simulink model "lf"  (Simulink 8.1)
settings: Solver=ode45  StartTime=0.0  StopTime=10.0  RelTol=1e-3
values from neighbouring files (symbols this model uses):
  A2 = 1.82742    [lf_param.m]
  A3 = 0.827764    [lf_param.m]
  B1 = 2.74759    [lf_param.m]
  B2 = 2.70322    [lf_param.m]
  fs = sq_wave_freq*osr    (= 10000)    [param2.m]
settings Model: Creator=amr  LastModifiedBy=amr
settings DataIOCC: SignalLoggingSaveFormat=Dataset
settings OptimizationCC: ExpressionDepthLimit=128
settings DebuggingCC: FcnCallInpInsideContextMsg=EnableAllAsError
settings GRTTargetCC: CombineOutputUpdateFcns=on  GRTInterface=off

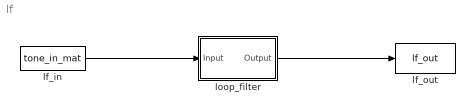
== system lf ==
  lf_in : FromWorkspace  VariableName=tone_in_mat  OutDataTypeStr=fixdt(1,16,15)  SampleTime=1/fs  Interpolate=off  OutputAfterFinalValue=Holding final value
  lf_out : ToWorkspace  VariableName=lf_out  SampleTime=-1
  loop_filter : Subsystem  Tag=FilterWizardSubSystem
      settings: ErrorFcn=dspFilterRealizedInBasicElemsAlgLoopErrFcnCallback
  wires:
  lf_in/1 -> loop_filter/1(Input)
  loop_filter/1(Output) -> lf_out/1

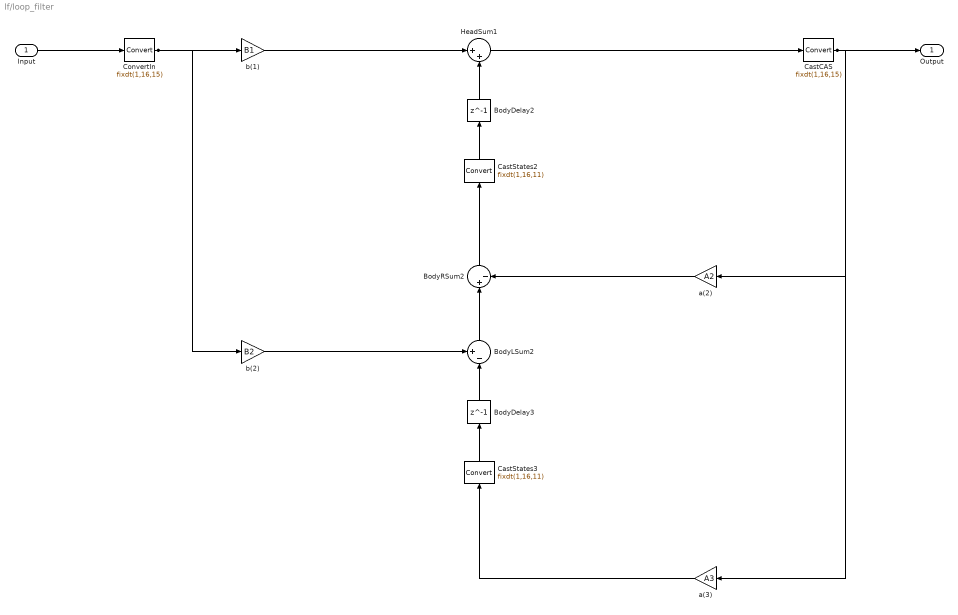
== system lf/loop_filter ==
  Input : Inport
  BodyDelay2 : Delay  DelayLength=1  InitialCondition=0
  BodyDelay3 : Delay  DelayLength=1  InitialCondition=0
  BodyLSum2 : Sum  Inputs=+-|  AccumDataTypeStr=fixdt(1,35,30)  OutDataTypeStr=fixdt(1,25,20)  SaturateOnIntegerOverflow=on
  BodyRSum2 : Sum  Inputs=|+-  AccumDataTypeStr=fixdt(1,35,30)  OutDataTypeStr=fixdt(1,25,20)  SaturateOnIntegerOverflow=on
  CastCAS : DataTypeConversion  OutDataTypeStr=fixdt(1,16,15)  SaturateOnIntegerOverflow=on
  CastStates2 : DataTypeConversion  OutDataTypeStr=fixdt(1,16,11)  SaturateOnIntegerOverflow=on
  CastStates3 : DataTypeConversion  OutDataTypeStr=fixdt(1,16,11)  SaturateOnIntegerOverflow=on
  ConvertIn : DataTypeConversion  OutDataTypeStr=fixdt(1,16,15)  RndMeth=Nearest  SaturateOnIntegerOverflow=on
  HeadSum1 : Sum  Inputs=|++  AccumDataTypeStr=fixdt(1,35,30)  OutDataTypeStr=fixdt(1,25,20)  SaturateOnIntegerOverflow=on
  a(2) : Gain  Gain=A2  ParamDataTypeStr=fixdt(1,16,14)  OutDataTypeStr=fixdt(1,25,22)  SaturateOnIntegerOverflow=on
  a(3) : Gain  Gain=A3  ParamDataTypeStr=fixdt(1,16,14)  OutDataTypeStr=fixdt(1,25,22)  SaturateOnIntegerOverflow=on
  b(1) : Gain  Gain=B1  ParamDataTypeStr=fixdt(1,16,15)  OutDataTypeStr=fixdt(1,25,24)  SaturateOnIntegerOverflow=on
  b(2) : Gain  Gain=B2  ParamDataTypeStr=fixdt(1,16,15)  OutDataTypeStr=fixdt(1,25,24)  SaturateOnIntegerOverflow=on
  Output : Outport
  wires:
  Input/1 -> ConvertIn/1
  b(1)/1 -> HeadSum1/1
  HeadSum1/1 -> CastCAS/1
  CastCAS/1 -> Output/1, a(2)/1, a(3)/1
  ConvertIn/1 -> b(1)/1, b(2)/1
  b(2)/1 -> BodyLSum2/1
  BodyLSum2/1 -> BodyRSum2/1
  BodyRSum2/1 -> CastStates2/1
  a(2)/1 -> BodyRSum2/2
  BodyDelay2/1 -> HeadSum1/2
  CastStates2/1 -> BodyDelay2/1
  a(3)/1 -> CastStates3/1
  BodyDelay3/1 -> BodyLSum2/2
  CastStates3/1 -> BodyDelay3/1
